simulink model "qraw_readDemo"  (R2016a)
settings: Solver=ode5  StartTime=0.0  StopTime=inf  FixedStep=0.001  RelTol=1e-3
libraries: dcpctrl x1
settings Model: SimulationMode=external  Creator=julianleland  LastModifiedBy=julianleland
settings HardwareCC: ProdBitPerLong=64  ProdLargestAtomicFloat=None  ProdHWDeviceType=Intel->x86-64  TargetBitPerLong=64  TargetBitPerPointer=64  TargetIntDivRoundTo=Zero  TargetEndianess=LittleEndian  TargetWordSize=64  TargetHWDeviceType=Intel->x86-64
settings RTWCC: SystemTargetFile=sldrt.tlc  TemplateMakefile=sldrt.tmf  Description=Simulink Desktop Real-Time  RTWCompilerOptimization=on
settings CodeAppCC: MaxIdLength=95
settings SimulinkDesktopRealTimeCC: TargetPreCompLibLocation=/Applications/MATLAB_R2016a.app/toolbox/sldrt/lib/maci64  TargetLangStandard=C89/C90 (ANSI)  SupportVariableSizeSignals=off

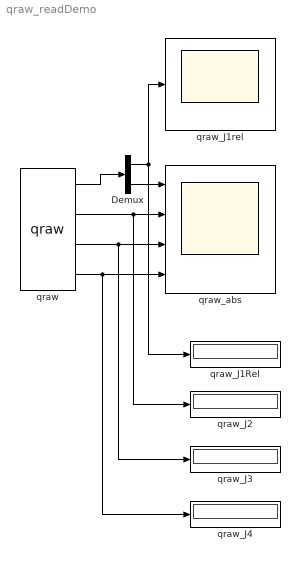
== system qraw_readDemo ==
  Demux : Demux  Outputs=2
  qraw : dcpctrl/qraw
  qraw_J1Rel : Display
  qraw_J1rel : Scope
  qraw_J2 : Display
  qraw_J3 : Display
  qraw_J4 : Display
  qraw_abs : Scope  NumInputPorts=4
  wires:
  qraw/1 -> Demux/1
  qraw/4 -> qraw_J4/1, qraw_abs/4
  qraw/3 -> qraw_J3/1, qraw_abs/3
  qraw/2 -> qraw_J2/1, qraw_abs/2
  Demux/2 -> qraw_abs/1
  Demux/1 -> qraw_J1rel/1, qraw_J1Rel/1
